simulink model "IO_mio_sim"  (R2023b)
settings: Solver=VariableStepAuto  StartTime=0.0  StopTime=10.0  RelTol=1e-3
values from neighbouring files (symbols this model uses):
  x0 = [3;5]    [IO_mio.m]
settings Model: Creator=stefa  LastModifiedBy=stefa

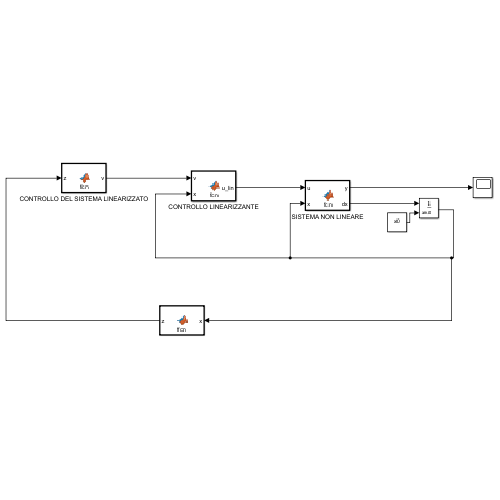
[thumbnail: Simulink's stored preview of the top-level diagram]
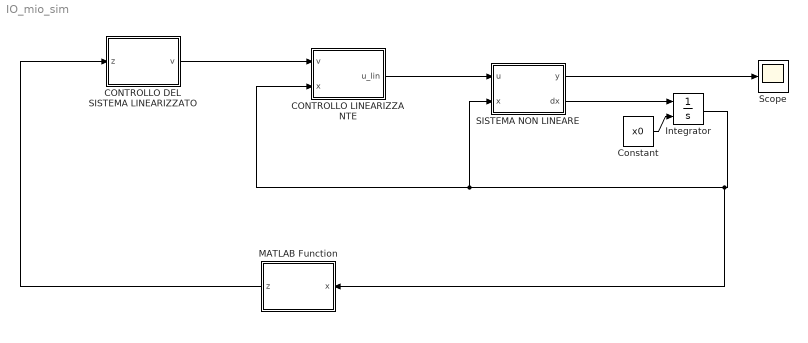
== system IO_mio_sim ==
  CONTROLLO DEL SISTEMA LINEARIZZATO : MATLAB Function  TreatAsAtomicUnit=on
  CONTROLLO LINEARIZZANTE : MATLAB Function  TreatAsAtomicUnit=on
  Constant : Constant  Value=x0
  Integrator : Integrator  InitialConditionSource=external
  MATLAB Function : MATLAB Function  TreatAsAtomicUnit=on
  SISTEMA NON LINEARE : MATLAB Function  TreatAsAtomicUnit=on
  Scope : Scope
  wires:
  SISTEMA NON LINEARE/2(dx) -> Integrator/1
  Integrator/1 -> MATLAB Function/1(x), CONTROLLO LINEARIZZANTE/2(x), SISTEMA NON LINEARE/2(x)
  Constant/1 -> Integrator/2
  CONTROLLO LINEARIZZANTE/1(u_lin) -> SISTEMA NON LINEARE/1(u)
  CONTROLLO DEL SISTEMA LINEARIZZATO/1(v) -> CONTROLLO LINEARIZZANTE/1(v)
  MATLAB Function/1(z) -> CONTROLLO DEL SISTEMA LINEARIZZATO/1(z)
  SISTEMA NON LINEARE/1(y) -> Scope/1

== matlab function IO_mio_sim/SISTEMA NON LINEARE ==
  data: u input; y output; x input; dx output
function [y,dx]= fcn(u,x)
x1=x(1);
x2=x(2);
dx=[(x1^2+x1)*x2;
    -2*x2+x1-x2*u+6*u];
y = 5*x1;

== matlab function IO_mio_sim/CONTROLLO DEL SISTEMA LINEARIZZATO ==
  data: z input; v output
function v = fcn(z)

v=-50*z(1)-15*z(2);

== matlab function IO_mio_sim/MATLAB Function ==
  data: x input; z output
function z = fcn(x)
x1=x(1);
x2=x(2);
z=[5*x1; 5*x2*(x1^2 + x1)];

== matlab function IO_mio_sim/CONTROLLO LINEARIZZANTE ==
  data: v input; u_lin output; x input
function u_lin = fcn(v,x)
x1=x(1);
x2=x(2);
u_lin=((5*x1^2 + 5*x1)*(x1 - 2*x2) - v + 5*x2^2*(2*x1 + 1)*(x1^2 + x1))/((5*x1^2 + 5*x1)*(x2 - 6));
